simulink model "s_rotpen_bal"  (Simulink 9.1)
settings: Solver=ode4  StartTime=0.0  StopTime=9  FixedStep=0.001  RelTol=1e-3  EnableMultiTasking=on
values from neighbouring files (symbols this model uses):
  A = [zeros(2), eye(2); disjointed_state]    [pendulum_arduino.m]
  B = [0; 0; disjointed_input]    [pendulum_arduino.m]
  C = eye(4)    [pendulum_arduino.m]
  D = zeros(4,1)    [pendulum_arduino.m]
  hpf_freq = 100    [pendulum_arduino.m]
  K = lqr(A,B,Q,R)    [pendulum_arduino.m]
libraries: simulink_extras x3
settings Model: Creator=MLevis  LastModifiedBy=Steve  ExtModeTrigDuration=10000
settings SolverCC: PositivePriorityOrder=on
settings DataIOCC: LimitDataPoints=on  SignalLoggingSaveFormat=ModelDataLogs
settings OptimizationCC: BooleanDataType=off  OptimizeBlockIOStorage=off  BufferReuse=off  GlobalBufferReuse=off  ExpressionFolding=off  ExpressionDepthLimit=2147483647  LocalBlockOutputs=off  InitFltsAndDblsToZero=on  OptimizeDataStoreBuffers=off  BusAssignmentInplaceUpdate=off
settings DebuggingCC: SaveWithParameterizedLinksMsg=none  SignalResolutionControl=TryResolveAllWithWarning  MultiTaskDSMMsg=warning  MultiTaskCondExecSysMsg=none  FcnCallInpInsideContextMsg=warning  StateNameClashWarn=warning
settings HardwareCC: TargetHWDeviceType=32-bit Generic
settings RTWCC: SystemTargetFile=quarc_windows.tlc  TemplateMakefile=quarc_default_tmf  Description=Quarc Win32 Target
settings STFCustomTargetCC: TargetFcnLib=ansi_tfl_tmw.mat  TargetPreCompLibLocation=C:\PROGRA~3\QUARC\lib\2014a\windows\release  GeneratePreprocessorConditionals=Disable all  CPPClassGenCompliant=on  SystemTargetFile=quarc_windows.tlc
settings GRTTargetCC: TargetFcnLib=ansi_tfl_tmw.mat  TargetPreCompLibLocation=C:\PROGRA~3\QUARC\lib\2014a\windows\release  ParMdlRefBuildCompliant=off  CompOptLevelCompliant=off  ConcurrentExecutionCompliant=off  GeneratePreprocessorConditionals=Disable all  MatFileLogging=off  UseToolchainInfoCompliant=off  ExtMode=on  ExtModeMexFile=quarc_comm
settings ConfigComp: CovSFcnEnable=off

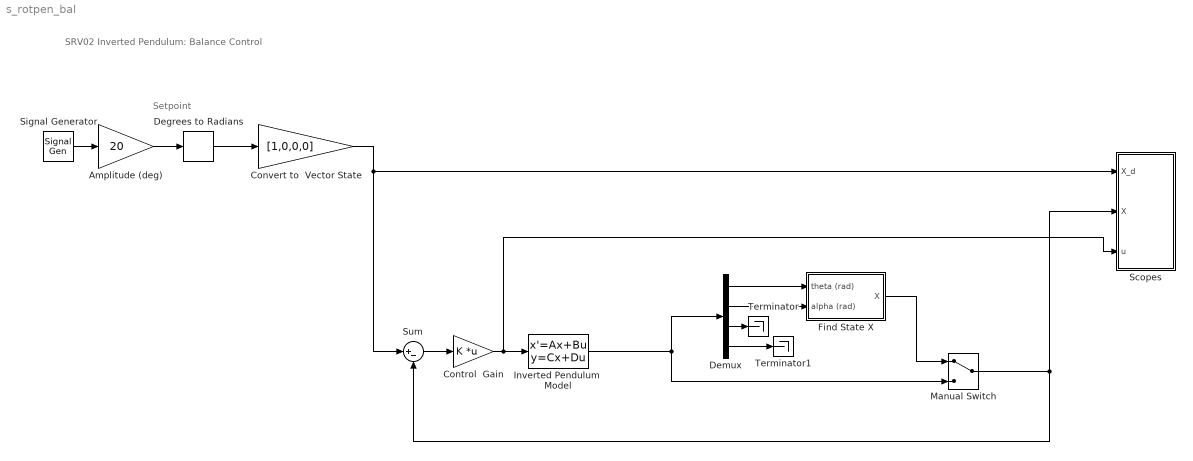
== system s_rotpen_bal ==
  note: Setpoint
  note: SRV02 Inverted Pendulum: Balance Control
  Amplitude (deg) : Gain  Gain=20  SaturateOnIntegerOverflow=on  OutDataTypeStr=Inherit: Same as input  ParamDataTypeStr=Inherit: Same as input
  Control  Gain : Gain  Gain=K  Multiplication=Matrix(K*u)
  Convert to  Vector State : Gain  Gain=[1,0,0,0]
  Degrees to Radians : simulink_extras/Transformations/Degrees to Radians
  Demux : Demux
  Find State X : Subsystem
  Inverted Pendulum  Model : StateSpace  A=A  B=B  C=C  D=D  InitialCondition=0
  Manual Switch : ManualSwitch
  Scopes : Subsystem
  Signal Generator : SignalGenerator  WaveForm=square  Frequency=0.1
  Sum : Sum  Inputs=|+-
  Terminator : Terminator
  Terminator1 : Terminator
  wires:
  Amplitude (deg)/1 -> Degrees to Radians/1
  Signal Generator/1 -> Amplitude (deg)/1
  Convert to  Vector State/1 -> Scopes/1(X_d), Sum/1
  Manual Switch/1 -> Scopes/2(X), Sum/2
  Sum/1 -> Control  Gain/1
  Control  Gain/1 -> Inverted Pendulum  Model/1, Scopes/3(u)
  Demux/1 -> Find State X/1(theta (rad))
  Demux/2 -> Find State X/2(alpha (rad))
  Degrees to Radians/1 -> Convert to  Vector State/1
  Inverted Pendulum  Model/1 -> Manual Switch/2, Demux/1
  Demux/3 -> Terminator/1
  Demux/4 -> Terminator1/1
  Find State X/1(X) -> Manual Switch/1

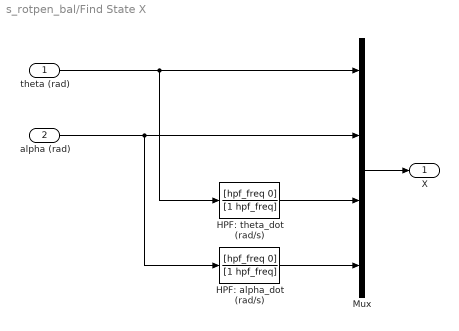
== system s_rotpen_bal/Find State X ==
  theta (rad) : Inport
  alpha (rad) : Inport  Port=2
  HPF: alpha_dot (rad/s) : TransferFcn  Numerator=[hpf_freq 0]  Denominator=[1 hpf_freq]
  HPF: theta_dot (rad/s) : TransferFcn  Numerator=[hpf_freq 0]  Denominator=[1 hpf_freq]
  Mux : Mux
  X : Outport
  wires:
  alpha (rad)/1 -> Mux/2, HPF: alpha_dot (rad/s)/1
  Mux/1 -> X/1
  theta (rad)/1 -> Mux/1, HPF: theta_dot (rad/s)/1
  HPF: theta_dot (rad/s)/1 -> Mux/3
  HPF: alpha_dot (rad/s)/1 -> Mux/4

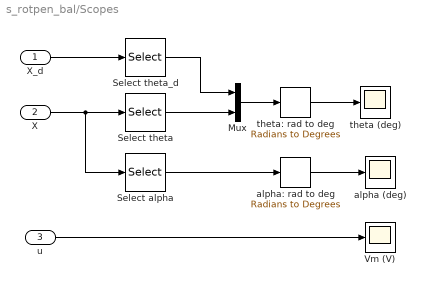
== system s_rotpen_bal/Scopes ==
  X_d : Inport
  X : Inport  Port=2
  u : Inport  Port=3
  Mux : Mux  Inputs=2
  Select alpha : Selector  InputPortWidth=4  IndexOptions=Index vector (dialog)  Indices=2  OutputSizes=[(-2)]
  Select theta : Selector  InputPortWidth=4  IndexOptions=Index vector (dialog)  Indices=1  OutputSizes=[(-2)]
  Select theta_d : Selector  InputPortWidth=4  IndexOptions=Index vector (dialog)  Indices=1  OutputSizes=[(-2)]
  Vm (V) : Scope
  alpha (deg) : Scope
  alpha: rad to deg : simulink_extras/Transformations/Radians to Degrees
  theta (deg) : Scope
  theta: rad to deg : simulink_extras/Transformations/Radians to Degrees
  wires:
  X_d/1 -> Select theta_d/1
  Select alpha/1 -> alpha: rad to deg/1
  X/1 -> Select alpha/1, Select theta/1
  Select theta_d/1 -> Mux/1
  Select theta/1 -> Mux/2
  u/1 -> Vm (V)/1
  alpha: rad to deg/1 -> alpha (deg)/1
  Mux/1 -> theta: rad to deg/1
  theta: rad to deg/1 -> theta (deg)/1
